simulink subsystem "Electrode_Hydraulic"  (R2025b)
settings: Solver=VariableStepAuto  StartTime=0.0  StopTime=10.0  RelTol=1e-3
settings Model: Creator=LYG  LastModifiedBy=i336

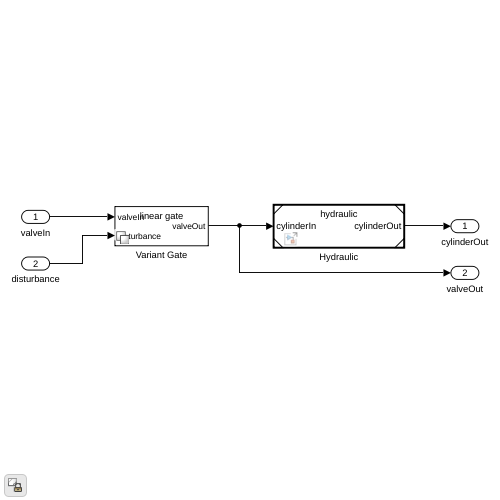
[thumbnail: Simulink's stored preview of the top-level diagram]
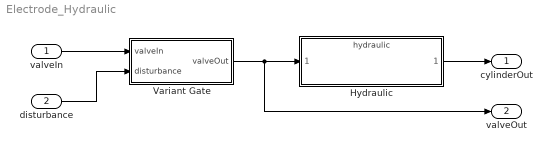
== system Electrode_Hydraulic ==
  valveIn : Inport
  disturbance : Inport  Port=2
  Hydraulic : ModelReference  ModelNameDialog=hydraulic.slx  SimulationMode=Normal  ModelReferenceVersion=3.16  Ap=Ap  Ct=Ct  Fforce=Fforce  Gmass=Gmass  Kc=Kc  Kq=Kq  Ve=Ve  beta_e=beta_e  L_init=L_init
  Variant Gate : Subsystem  Variant=on
  cylinderOut : Outport
  valveOut : Outport  Port=2
  wires:
  Hydraulic/1 -> cylinderOut/1
  valveIn/1 -> Variant Gate/1(valveIn)
  Variant Gate/1(valveOut) -> Hydraulic/1, valveOut/1
  disturbance/1 -> Variant Gate/2(disturbance)

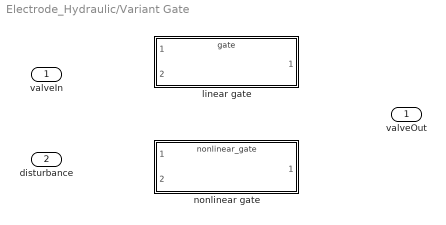
== system Electrode_Hydraulic/Variant Gate ==
  valveIn : Inport
  disturbance : Inport  Port=2
  linear gate : ModelReference  ModelNameDialog=gate.slx  SimulationMode=Normal  VariantControl=GateChoice == 'linear'  ModelReferenceVersion=3.12
  nonlinear gate : ModelReference  ModelNameDialog=nonlinear_gate.slx  SimulationMode=Normal  VariantControl=GateChoice == 'nonlinear'  ModelReferenceVersion=1.12
  valveOut : Outport
